simulink model "FM_modulation_discrete"  (R2023b)
settings: Solver=ode45  StartTime=0.0  StopTime=0.5  RelTol=1e-3  EnableMultiTasking=on
settings Model: Creator=mm  LastModifiedBy=Anu
settings SolverCC: AlgebraicLoopSolver=TrustRegion
settings DataIOCC: LimitDataPoints=on  SaveFormat=Array  ReturnWorkspaceOutputs=off
settings OptimizationCC: LifeSpan=inf
settings DebuggingCC: SolverPrmCheckMsg=warning  UnconnectedInputMsg=warning  UnconnectedOutputMsg=warning  UnconnectedLineMsg=warning  SFUnexpectedBacktrackingDiag=warning  SFNoUnconditionalDefaultTransitionDiag=warning  SFExecutionAtInitializationDiag=none  ArithmeticOperatorsInVariantConditions=warning
settings HardwareCC: ProdBitPerPointer=32  ProdBitPerSizeT=32  ProdBitPerPtrDiffT=32  ProdLargestAtomicFloat=None  ProdIntDivRoundTo=Undefined  ProdEndianess=Unspecified  ProdWordSize=32  ProdHWDeviceType=32-bit Generic
settings ModelReferenceCC: PropagateSignalLabelsOutOfModel=off
settings SFSimCC: SimUseLocalCustomCode=off  CustomCodeUndefinedFunction=UseInterfaceOnly
settings RTWCC: RTWUseLocalCustomCode=off
settings CodeAppCC: StateflowObjectComments=on
settings GRTTargetCC: TargetLangStandard=C89/C90 (ANSI)
settings ConfigComp: CovMetricSettings=dw  CovSaveCumulativeToWorkspaceVar=on  CovSaveSingleToWorkspaceVar=on  CovExternalEMLEnable=off  CovSFcnEnable=off

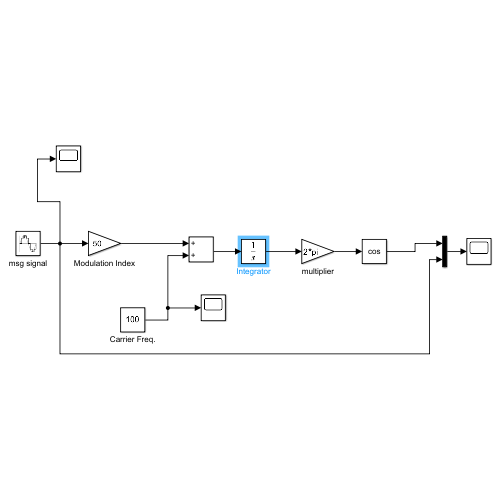
[thumbnail: Simulink's stored preview of the top-level diagram]
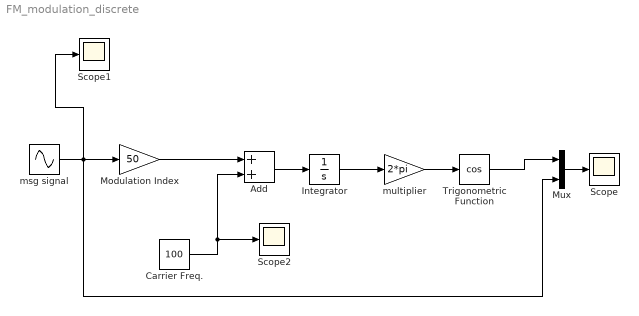
== system FM_modulation_discrete ==
  Add : Sum
  Carrier Freq. : Constant  Value=100
  Integrator : Integrator
  Modulation Index : Gain  Gain=50
  Mux : Mux  Inputs=2
  Scope : Scope
  Scope1 : Scope
  Scope2 : Scope
  Trigonometric Function : Trigonometry  Operator=cos
  msg signal : Sin  Frequency=2*pi*10  SampleTime=0.0001
  multiplier : Gain  Gain=2*pi
  wires:
  msg signal/1 -> Scope1/1, Mux/2, Modulation Index/1
  Modulation Index/1 -> Add/1
  Carrier Freq./1 -> Add/2, Scope2/1
  Add/1 -> Integrator/1
  Integrator/1 -> multiplier/1
  multiplier/1 -> Trigonometric Function/1
  Mux/1 -> Scope/1
  Trigonometric Function/1 -> Mux/1
